simulink model "System"  (R2019b)
settings: Solver=VariableStepAuto  StartTime=0.0  StopTime=10.0  RelTol=1e-3
PreLoadFcn:
  | load AllBuses
settings Model: Creator=Lenovo  LastModifiedBy=Lenovo
settings OptimizationCC: DefaultParameterBehavior=Inlined

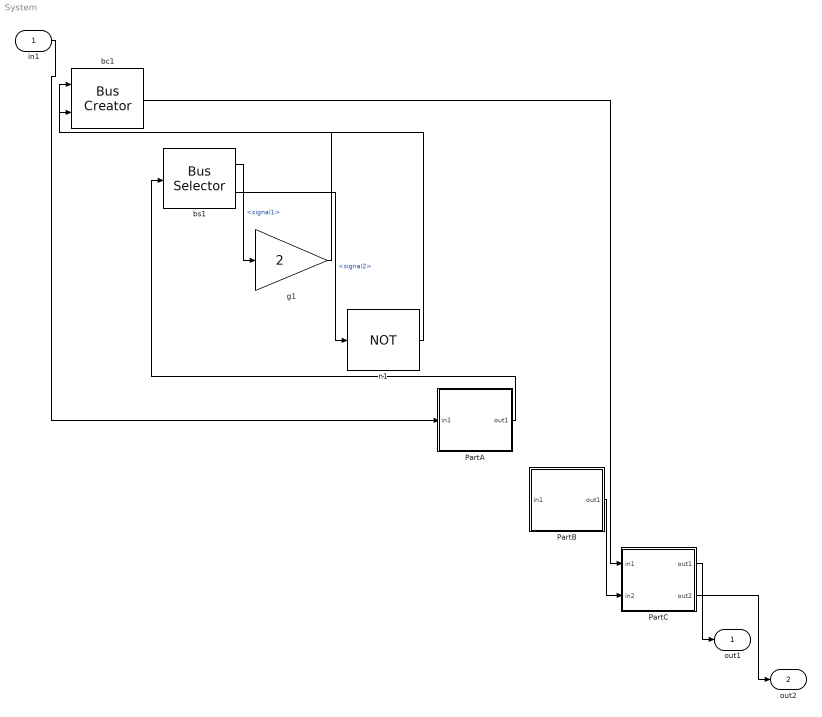
== system System ==
  in1 : Inport  OutDataTypeStr=Bus: Bus_1  BusOutputAsStruct=on
  PartA : Subsystem
  PartB : Subsystem
  PartC : Subsystem
  bc1 : BusCreator  Inputs=2  OutDataTypeStr=Bus: Bus_1  NonVirtualBus=on
  bs1 : BusSelector  OutputSignals=signal1,signal2
  g1 : Gain  Gain=2  SaturateOnIntegerOverflow=on  OutDataTypeStr=Inherit: Same as input  ParamDataTypeStr=Inherit: Same as input
  n1 : Logic  Operator=NOT
  out1 : Outport  OutDataTypeStr=Bus: Bus_1  BusOutputAsStruct=on
  out2 : Outport  Port=2  OutDataTypeStr=Bus: Bus_3  BusOutputAsStruct=on
  wires:
  bc1/1 -> PartC/1(in1)
  bs1/1 -> g1/1  "<signal1>"
  bs1/2 -> n1/1  "<signal2>"
  g1/1 -> bc1/1
  in1/1 -> PartA/1(in1)
  n1/1 -> bc1/2
  PartA/1(out1) -> bs1/1
  PartB/1(out1) -> PartC/2(in2)
  PartC/1(out1) -> out1/1
  PartC/2(out2) -> out2/1

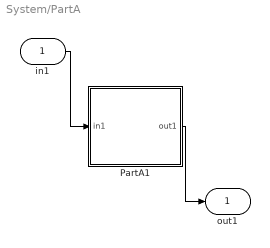
== system System/PartA ==
  in1 : Inport  OutDataTypeStr=Bus: Bus_1  BusOutputAsStruct=on
  PartA1 : Subsystem
  out1 : Outport  OutDataTypeStr=Bus: Bus_1  BusOutputAsStruct=on
  wires:
  in1/1 -> PartA1/1(in1)
  PartA1/1(out1) -> out1/1

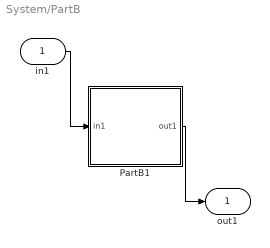
== system System/PartB ==
  in1 : Inport  OutDataTypeStr=Bus: Bus_2  BusOutputAsStruct=on
  PartB1 : Subsystem
  out1 : Outport  OutDataTypeStr=Bus: Bus_2  BusOutputAsStruct=on
  wires:
  in1/1 -> PartB1/1(in1)
  PartB1/1(out1) -> out1/1

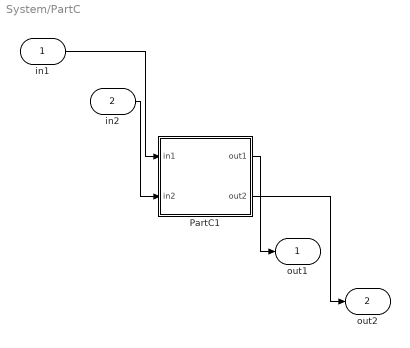
== system System/PartC ==
  in1 : Inport  OutDataTypeStr=Bus: Bus_1  BusOutputAsStruct=on
  in2 : Inport  Port=2  OutDataTypeStr=Bus: Bus_2  BusOutputAsStruct=on
  PartC1 : Subsystem
  out1 : Outport  OutDataTypeStr=Bus: Bus_1  BusOutputAsStruct=on
  out2 : Outport  Port=2  OutDataTypeStr=Bus: Bus_3  BusOutputAsStruct=on
  wires:
  in1/1 -> PartC1/1(in1)
  in2/1 -> PartC1/2(in2)
  PartC1/1(out1) -> out1/1
  PartC1/2(out2) -> out2/1

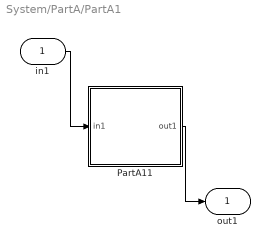
== system System/PartA/PartA1 ==
  in1 : Inport  OutDataTypeStr=Bus: Bus_1  BusOutputAsStruct=on
  PartA11 : Subsystem
  out1 : Outport  OutDataTypeStr=Bus: Bus_1  BusOutputAsStruct=on
  wires:
  in1/1 -> PartA11/1(in1)
  PartA11/1(out1) -> out1/1

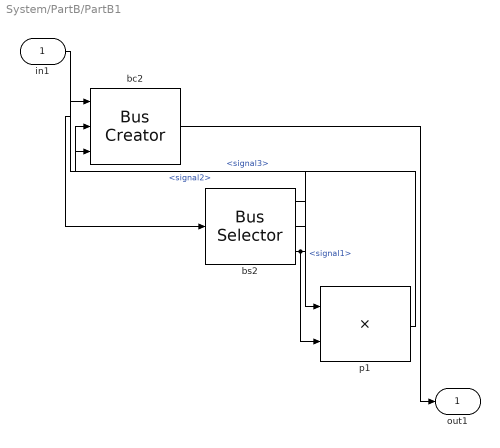
== system System/PartB/PartB1 ==
  in1 : Inport  OutDataTypeStr=Bus: Bus_2  BusOutputAsStruct=on
  bc2 : BusCreator  Inputs=3  OutDataTypeStr=Bus: Bus_2  NonVirtualBus=on
  bs2 : BusSelector  OutputSignals=signal1,signal2,signal3
  p1 : Product  Inputs=**  SaturateOnIntegerOverflow=on  RndMeth=Zero  OutDataTypeStr=Inherit: Same as first input
  out1 : Outport  OutDataTypeStr=Bus: Bus_2  BusOutputAsStruct=on
  wires:
  bc2/1 -> out1/1
  bs2/1 -> p1/1  "<signal1>"
  bs2/2 -> bc2/2  "<signal2>"
  bs2/3 -> bc2/3, p1/2  "<signal3>"
  in1/1 -> bs2/1
  p1/1 -> bc2/1

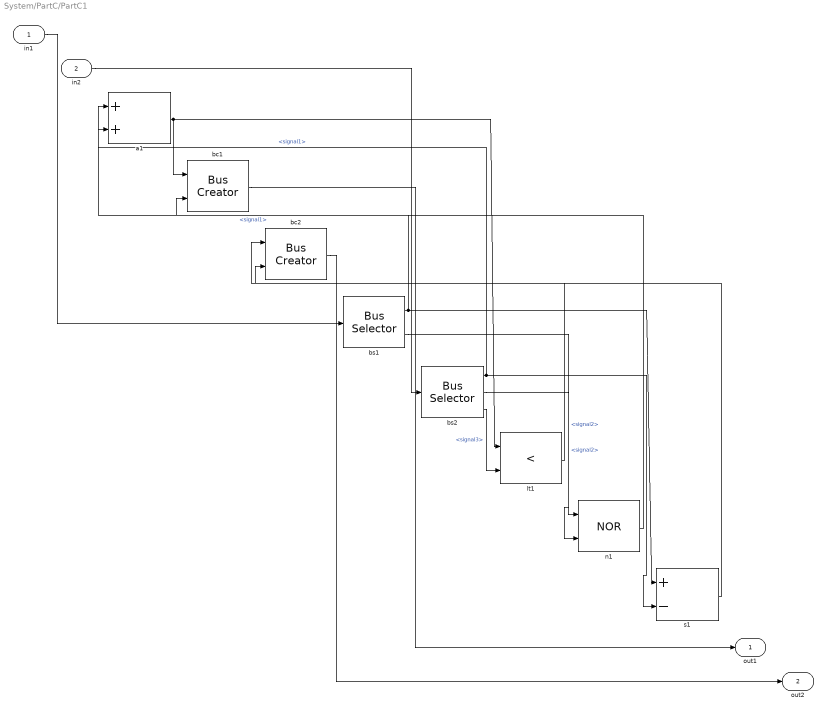
== system System/PartC/PartC1 ==
  in1 : Inport  OutDataTypeStr=Bus: Bus_1  BusOutputAsStruct=on
  in2 : Inport  Port=2  OutDataTypeStr=Bus: Bus_2  BusOutputAsStruct=on
  a1 : Sum  SaturateOnIntegerOverflow=on  InputSameDT=on  OutDataTypeStr=Inherit: Same as first input
  bc1 : BusCreator  Inputs=2  OutDataTypeStr=Bus: Bus_1  NonVirtualBus=on
  bc2 : BusCreator  Inputs=2  OutDataTypeStr=Bus: Bus_3  NonVirtualBus=on
  bs1 : BusSelector  OutputSignals=signal1,signal2
  bs2 : BusSelector  OutputSignals=signal1,signal2,signal3
  lt1 : RelationalOperator  Operator=<  RndMeth=Nearest
  n1 : Logic  Operator=NOR
  s1 : Sum  Inputs=+-  SaturateOnIntegerOverflow=on  InputSameDT=on  OutDataTypeStr=Inherit: Same as first input
  out1 : Outport  OutDataTypeStr=Bus: Bus_1  BusOutputAsStruct=on
  out2 : Outport  Port=2  OutDataTypeStr=Bus: Bus_3  BusOutputAsStruct=on
  wires:
  a1/1 -> bc1/1, lt1/1
  bc1/1 -> out1/1
  bc2/1 -> out2/1
  bs1/1 -> a1/1, s1/1  "<signal1>"
  bs1/2 -> n1/1  "<signal2>"
  bs2/1 -> a1/2, s1/2  "<signal1>"
  bs2/2 -> n1/2  "<signal2>"
  bs2/3 -> lt1/2  "<signal3>"
  in1/1 -> bs1/1
  in2/1 -> bs2/1
  lt1/1 -> bc2/2
  n1/1 -> bc1/2
  s1/1 -> bc2/1

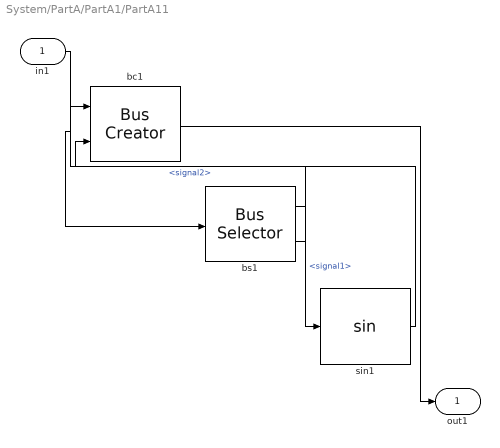
== system System/PartA/PartA1/PartA11 ==
  in1 : Inport  OutDataTypeStr=Bus: Bus_1  BusOutputAsStruct=on
  bc1 : BusCreator  Inputs=2  OutDataTypeStr=Bus: Bus_1  NonVirtualBus=on
  bs1 : BusSelector  OutputSignals=signal1,signal2
  sin1 : Trigonometry
  out1 : Outport  OutDataTypeStr=Bus: Bus_1  BusOutputAsStruct=on
  wires:
  bc1/1 -> out1/1
  bs1/1 -> sin1/1  "<signal1>"
  bs1/2 -> bc1/2  "<signal2>"
  in1/1 -> bs1/1
  sin1/1 -> bc1/1
